simulink model "convert_voltagesignal_to_currentsignal"  (R2022b)
settings: Solver=VariableStepAuto  StartTime=0.0  StopTime=10.0  MaxStep=1e-3  RelTol=1e-3
settings Model: Creator=Dell  LastModifiedBy=Dell

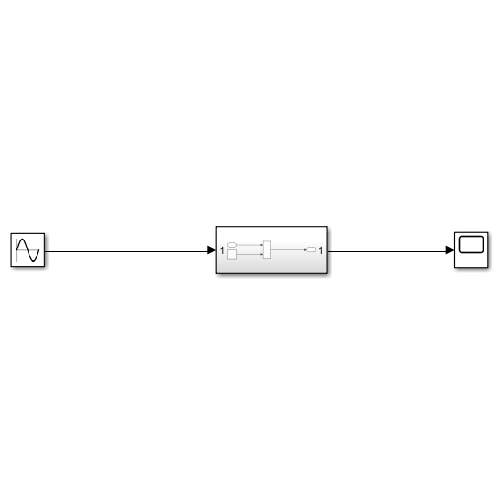
[thumbnail: Simulink's stored preview of the top-level diagram]
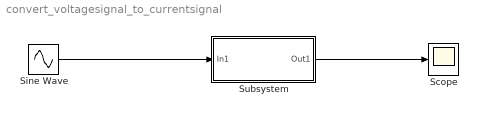
== system convert_voltagesignal_to_currentsignal ==
  Scope : Scope
  Sine Wave : Sin  Amplitude=220  Frequency=2*pi*50  SampleTime=0
  Subsystem : Subsystem
  wires:
  Sine Wave/1 -> Subsystem/1(In1)
  Subsystem/1(Out1) -> Scope/1

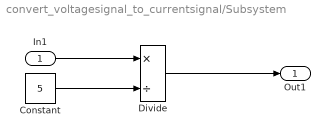
== system convert_voltagesignal_to_currentsignal/Subsystem ==
  In1 : Inport
  Constant : Constant  Value=5
  Divide : Product  Inputs=*/
  Out1 : Outport
  wires:
  In1/1 -> Divide/1
  Constant/1 -> Divide/2
  Divide/1 -> Out1/1
